simulink model "Model_2"  (R2020b)
settings: Solver=VariableStepAuto  StartTime=0.0  StopTime=inf  RelTol=1e-3
settings Model: EnablePacing=on  Creator=Akarsh  LastModifiedBy=Akarsh

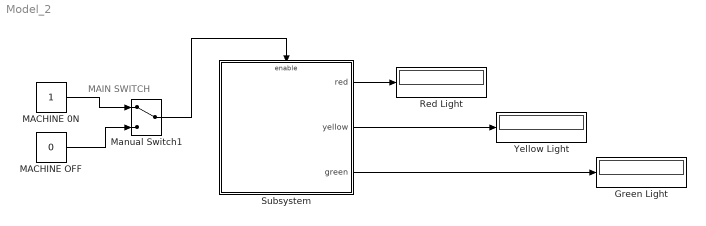
== system Model_2 ==
  note: MAIN SWITCH
  Green Light : Display
  MACHINE 0N : Constant
  MACHINE OFF : Constant  Value=0
  Manual Switch1 : ManualSwitch
  Red Light : Display
  Subsystem : Subsystem
  Yellow Light : Display
  wires:
  MACHINE OFF/1 -> Manual Switch1/2
  MACHINE 0N/1 -> Manual Switch1/1
  Subsystem/1(red) -> Red Light/1
  Subsystem/2(yellow) -> Yellow Light/1
  Subsystem/3(green) -> Green Light/1
  Manual Switch1/1 -> Subsystem/Enable

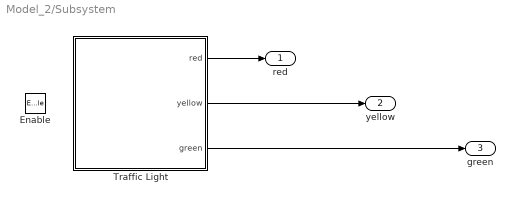
== system Model_2/Subsystem ==
  Enable : EnablePort
  "Traffic Light " : Stateflow chart  TreatAsAtomicUnit=on
  red : Outport
  yellow : Outport  Port=2
  green : Outport  Port=3
  wires:
  "Traffic Light "/1(red) -> red/1
  "Traffic Light "/3(green) -> green/1
  "Traffic Light "/2(yellow) -> yellow/1

== stateflow chart Model_2/Subsystem/Traffic Light  ==
  state Go
    entry:
    red=0;
    yellow=0;
    green=1;
  state prepareTostop
    entry:
    red=0;
    yellow=1;
    green=0;
  state Stop
    entry:
    red=1;
    yellow=0;
    green=0;
  (default) -> Stop
  Stop -> prepareTostop : after(10,sec)
  prepareTostop -> Go : after(2,sec)
  Go -> Stop : after(15,sec)
  data: red output =1; yellow output =0; green output =0
